simulink model "adcs_sim_main"  (R2016b)
settings: Solver=VariableStepAuto  StartTime=0.0  StopTime=60  RelTol=1e-3  EnableMultiTasking=on
libraries: actuators_lib x1, dynamics_lib x1, environment_lib x1, adcs_fsw_main x1, sensors_lib x1
settings Model: Creator=bbarz_000  LastModifiedBy=Sean
settings OptimizationCC: DefaultParameterBehavior=Inlined  UseDivisionForNetSlopeComputation=on  UseFloatMulNetSlope=on  InlineInvariantSignals=on  PassReuseOutputArgsAs=Individual arguments  ZeroExternalMemoryAtStartup=off  ZeroInternalMemoryAtStartup=off  NoFixptDivByZeroProtection=on  EfficientFloat2IntCast=on  LifeSpan=1
settings DebuggingCC: ParameterTunabilityLossMsg=error  SFUnexpectedBacktrackingDiag=warning  SFNoUnconditionalDefaultTransitionDiag=warning  SFExecutionAtInitializationDiag=none
settings HardwareCC: ProdBitPerInt=16  ProdBitPerPointer=16  ProdBitPerSizeT=16  ProdBitPerPtrDiffT=16  ProdLargestAtomicFloat=None  ProdWordSize=16  ProdHWDeviceType=Texas Instruments->MSP430
settings RTWCC: SystemTargetFile=ert.tlc  GenCodeOnly=on  TemplateMakefile=ert_default_tmf  Description=Embedded Coder  GenerateReport=on  IncludeHyperlinkInReport=on  LaunchReport=on  GenerateTraceInfo=on  GenerateTraceReport=on  GenerateTraceReportSl=on  GenerateTraceReportSf=on  GenerateTraceReportEml=on  GenerateCodeMetricsReport=on
settings CodeAppCC: ForceParamTrailComments=on  IgnoreCustomStorageClasses=off  OperatorAnnotations=on  SimulinkDataObjDesc=on  SFDataObjDesc=on  MATLABFcnDesc=on  CustomSymbolStrGlobalVar=rt$N$M  CustomSymbolStrType=$N$M  CustomSymbolStrFcn=$N$M$F  CustomSymbolStrMacro=$N$M  InsertBlockDesc=on  MATLABSourceComments=on
settings ERTTargetCC: GenerateSampleERTMain=on  CombineSignalStateStructs=on  SupportComplex=off  SupportContinuousTime=on  SupportNonInlinedSFcns=on  InlinedParameterPlacement=NonHierarchical  ERTCustomFileTemplate=example_file_process.tlc  ERTFilePackagingFormat=CompactWithDataFile
settings ConfigComp: CovMetricSettings=dw  CovHtmlReporting=on  CovSaveCumulativeToWorkspaceVar=on  CovSaveSingleToWorkspaceVar=on  CovExternalEMLEnable=off

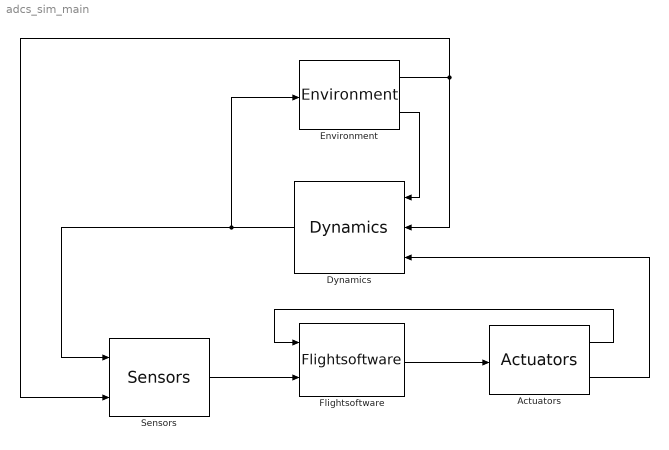
== system adcs_sim_main ==
  Actuators : actuators_lib/Actuators
  Dynamics : dynamics_lib/Dynamics
  Environment : environment_lib/Environment
  Flightsoftware : adcs_fsw_main/Flightsoftware
  Sensors : sensors_lib/Sensors
  wires:
  Flightsoftware/1 -> Actuators/1
  Dynamics/1 -> Environment/1, Sensors/1
  Sensors/1 -> Flightsoftware/2
  Environment/1 -> Sensors/2, Dynamics/2
  Actuators/2 -> Dynamics/3
  Actuators/1 -> Flightsoftware/1
  Environment/2 -> Dynamics/1
